simulink model "CACC_Center"  (R2022b)
settings: Solver=FixedStepAuto  StartTime=0.0  StopTime=Tsim  FixedStep=0.05  RelTol=1e-3
values from neighbouring files (symbols this model uses):
  h = 1.0    (= 1)    [ros_cacc.m]    (also in ros_cacc2.m)
  k1 = 1    [ros_cacc.m]    (also in ros_cacc2.m)
  k2 = 1    [ros_cacc.m]    (also in ros_cacc2.m)
  L = 0.32    [ros_cacc.m]    (also in ros_cacc2.m)
  r = 1    [ros_cacc.m]    (also in ros_cacc2.m)
  v_threshold = v_thr    (= 0.1)    [ros_cacc.m]    (also in ros_cacc2.m)
undefined symbols (not defined in the file or in its folder): angular, linear
libraries: ros2lib x7, robotcorelib x1
settings Model: VariantFading=off  Creator=harun  LastModifiedBy=harun
settings DataIOCC: ReturnWorkspaceOutputs=off
settings OptimizationCC: EnhancedBackFolding=on  PassReuseOutputArgsAs=Individual arguments  ZeroExternalMemoryAtStartup=off  ZeroInternalMemoryAtStartup=off  MaxStackSize=64  OptimizeBlockOrder=speed  DifferentSizesBufferReuse=on  OptimizationCustomize=off  EfficientTunableParamExpr=on
settings DebuggingCC: ParameterTunabilityLossMsg=error  UnconnectedInputMsg=warning  UnconnectedOutputMsg=warning  UnconnectedLineMsg=warning
settings HardwareCC: ProdBitPerLong=64  ProdHWDeviceType=Intel->x86-64 (Linux 64)
settings ModelReferenceCC: EnableRefExpFcnMdlSchedulingChecks=on
settings SFSimCC: MATLABDynamicMemAlloc=off
settings RTWCC: Description=Embedded Coder  SystemTargetFile=ert.tlc  HardwareBoard=Robot Operating System 2 (ROS 2)  TLCOptions="-aInlineSetEventsForThisBaseRateFcn=TLC_FALSE -aSuppressMultiTaskScheduler=TLC_FALSE  -aRateBasedStepFcn=0"  TemplateMakefile=ert_default_tmf  Toolchain=Colcon Tools  TargetLang=C++  DLArmComputeVersion=19.05
settings CodeAppCC: ForceParamTrailComments=on  IgnoreCustomStorageClasses=off  OperatorAnnotations=on  SimulinkDataObjDesc=on  SFDataObjDesc=on  InsertBlockDesc=on
settings ERTTargetCC: CodeInterfacePackaging=C++ class  SupportContinuousTime=on  SupportVariableSizeSignals=on  RootIOFormat=Structure reference

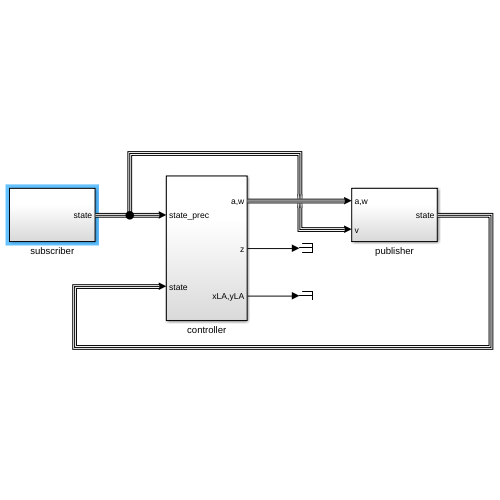
[thumbnail: Simulink's stored preview of the top-level diagram]
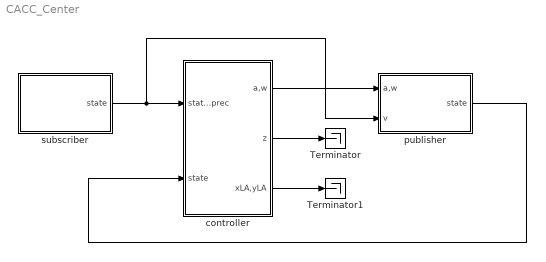
== system CACC_Center ==
  Terminator : Terminator
  Terminator1 : Terminator
  controller : Subsystem
  publisher : Subsystem
  subscriber : Subsystem
  wires:
  controller/3(xLA,yLA) -> Terminator1/1
  subscriber/1(state) -> publisher/2(v), controller/1(state_prec)
  publisher/1(state) -> controller/2(state)
  controller/1(a,w) -> publisher/1(a,w)
  controller/2(z) -> Terminator/1

== system CACC_Center/controller ==
  state_prec : Inport
  state : Inport  Port=2
  LA : Subsystem  TreatAsAtomicUnit=on
  a,w : Outport  VectorParamsAs1DForOutWhenUnconnected=off
  z : Outport  Port=2  VectorParamsAs1DForOutWhenUnconnected=off
  xLA,yLA : Outport  Port=3  VectorParamsAs1DForOutWhenUnconnected=off
  wires:
  state_prec/1 -> LA/1(state_prec)
  state/1 -> LA/2(state)
  LA/1(a,w) -> a,w/1
  LA/2(z) -> z/1
  LA/3(lookahead point) -> xLA,yLA/1

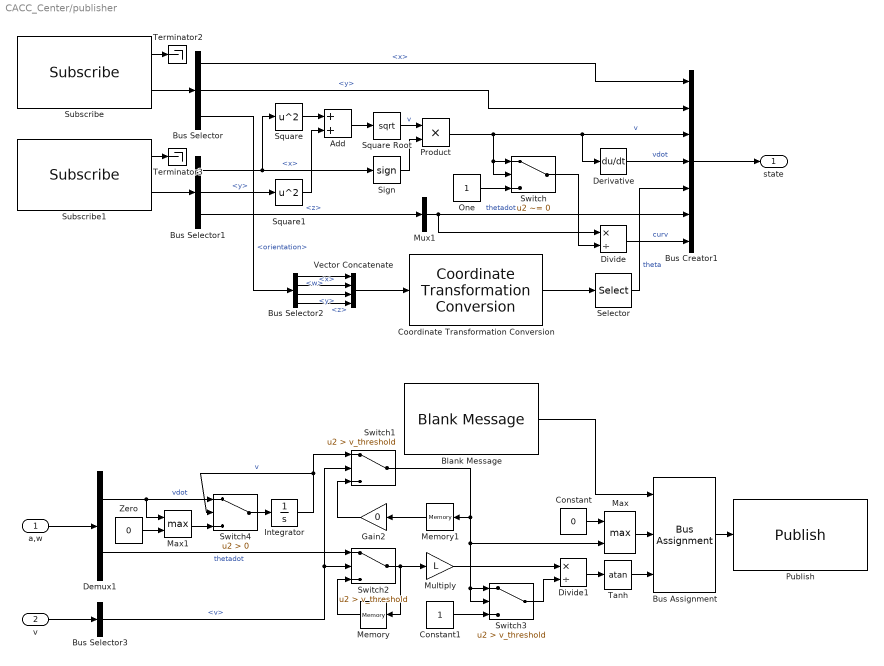
== system CACC_Center/publisher ==
  a,w : Inport
  v : Inport  Port=2
  Add : Sum
  Blank Message : ros2lib/Blank Message  messageClass=Message  entityType=geometry_msgs/Twist  messageType=geometry_msgs/Twist  SampleTime=0.05
  Bus Assignment : BusAssignment  AssignedSignals=linear.x,angular.z
  Bus Creator1 : BusCreator  Inputs=7
  Bus Selector : BusSelector  OutputSignals=pose.position.x,pose.position.y,pose.orientation
  Bus Selector1 : BusSelector  OutputSignals=twist.twist.linear.x,twist.twist.linear.y,twist.twist.angular.z
  Bus Selector2 : BusSelector  OutputSignals=w,x,y,z
  Bus Selector3 : BusSelector  OutputSignals=v
  Constant : Constant  Value=0
  Constant1 : Constant
  Coordinate Transformation Conversion : robotcorelib/Coordinate Transformation Conversion  InputRepresentation=Quaternion  InputEulerSequence=ZYX  ShowTrVecInputPort=on  OutputRepresentation=Euler Angles  OutputEulerSequence=ZYX  ShowTrVecOutputPort=on  SimulateUsing=Interpreted execution
  Demux1 : Demux  Outputs=2
  Derivative : Derivative
  Divide : Product  Inputs=*/
  Divide1 : Product  Inputs=*/
  Gain2 : Gain  Gain=0
  Integrator : Integrator  InitialCondition=0.0
  Max : MinMax  Function=max  Inputs=2
  Max1 : MinMax  Function=max  Inputs=2
  Memory : Memory
  Memory1 : Memory
  Multiply : Gain  Gain=L
  Mux1 : Mux  Inputs=1
  One : Constant  OutDataTypeStr=Inherit: Inherit via back propagation
  Product : Product
  Publish : ros2lib/Publish  topicSource=Specify your own  topic=cmd_vel  messageType=geometry_msgs/Twist  QOSHistory=Keep last  QOSDepth=1  QOSReliability=Reliable  QOSDurability=Volatile
  Selector : Selector  InputPortWidth=3  IndexOptions=Index vector (dialog)  Indices=[1]  OutputSizes=1
  Sign : Signum
  Square : Math  Operator=square
  Square Root : Sqrt
  Square1 : Math  Operator=square
  Subscribe : ros2lib/Subscribe  topicSource=Specify your own  topic=localization_pose  messageType=geometry_msgs/PoseStamped  sampleTime=0.1  QOSHistory=Keep last  QOSDepth=1  QOSReliability=Reliable  QOSDurability=Volatile
  Subscribe1 : ros2lib/Subscribe  topicSource=Specify your own  topic=odom  messageType=nav_msgs/Odometry  sampleTime=0.1  QOSHistory=Keep last  QOSDepth=1  QOSReliability=Reliable  QOSDurability=Volatile
  Switch : Switch  Criteria=u2 ~= 0  SaturateOnIntegerOverflow=off  InputSameDT=off
  Switch1 : Switch  Criteria=u2 > Threshold  Threshold=v_threshold  SaturateOnIntegerOverflow=off  InputSameDT=off
  Switch2 : Switch  Criteria=u2 > Threshold  Threshold=v_threshold  SaturateOnIntegerOverflow=off  InputSameDT=off
  Switch3 : Switch  Criteria=u2 > Threshold  Threshold=v_threshold  SaturateOnIntegerOverflow=off  InputSameDT=off
  Switch4 : Switch  Criteria=u2 > Threshold  SaturateOnIntegerOverflow=off  InputSameDT=off
  Tanh : Trigonometry  Operator=atan
  Terminator2 : Terminator
  Terminator3 : Terminator
  Vector Concatenate : Concatenate  NumInputs=4
  Zero : Constant  Value=0  OutDataTypeStr=Inherit: Inherit via back propagation
  state : Outport  VectorParamsAs1DForOutWhenUnconnected=off
  wires:
  Divide1/1 -> Tanh/1
  Mux1/1 -> Divide/1, Bus Creator1/6  "thetadot"
  Subscribe/1 -> Terminator2/1
  Subscribe/2 -> Bus Selector/1
  Subscribe1/2 -> Bus Selector1/1
  Subscribe1/1 -> Terminator3/1
  Memory1/1 -> Gain2/1
  Demux1/2 -> Switch2/1  "thetadot"
  Switch3/1 -> Divide1/2
  Memory/1 -> Switch2/3
  Switch/1 -> Divide/2
  Zero/1 -> Max1/2
  Divide/1 -> Bus Creator1/7  "curv"
  Selector/1 -> Bus Creator1/5  "theta"
  Switch2/1 -> Multiply/1, Memory/1
  Max1/1 -> Switch4/3
  Derivative/1 -> Bus Creator1/4  "vdot"
  Add/1 -> Square Root/1
  Integrator/1 -> Switch1/1, Switch4/2  "v"
  Bus Selector1/1 -> Square/1, Sign/1  "<x>"
  Square1/1 -> Add/2
  Square Root/1 -> Product/1  "v"
  Max/1 -> Bus Assignment/2
  Coordinate Transformation Conversion/1 -> Selector/1
  a,w/1 -> Demux1/1
  Bus Selector2/2 -> Vector Concatenate/2  "<x>"
  Product/1 -> Switch/1, Switch/2, Derivative/1, Bus Creator1/3  "v"
  Constant1/1 -> Switch3/3
  Bus Selector1/3 -> Mux1/1  "<z>"
  Demux1/1 -> Max1/1, Switch4/1  "vdot"
  Sign/1 -> Product/2
  Bus Selector2/1 -> Vector Concatenate/1  "<w>"
  Bus Assignment/1 -> Publish/1
  Bus Creator1/1 -> state/1
  Tanh/1 -> Bus Assignment/3
  Gain2/1 -> Switch1/3
  Blank Message/1 -> Bus Assignment/1
  Switch4/1 -> Integrator/1
  Bus Selector2/3 -> Vector Concatenate/3  "<y>"
  Switch1/1 -> Max/2, Switch3/1, Switch3/2, Memory1/1
  Vector Concatenate/1 -> Coordinate Transformation Conversion/1
  Bus Selector/3 -> Bus Selector2/1  "<orientation>"
  Constant/1 -> Max/1
  Square/1 -> Add/1
  Bus Selector/2 -> Bus Creator1/2  "<y>"
  Bus Selector3/1 -> Switch2/2, Switch1/2  "<v>"
  Bus Selector/1 -> Bus Creator1/1  "<x>"
  Bus Selector1/2 -> Square1/1  "<y>"
  One/1 -> Switch/3
  v/1 -> Bus Selector3/1
  Multiply/1 -> Divide1/1
  Bus Selector2/4 -> Vector Concatenate/4  "<z>"

== system CACC_Center/subscriber ==
  Bus Creator : BusCreator  Inputs=7
  Bus Selector : BusSelector  OutputSignals=x,y,v,vdot,theta,thetadot
  Derivative2 : Derivative
  Divide : Product  Inputs=*/
  One : Constant  OutDataTypeStr=Inherit: Inherit via back propagation
  Subscribe : ros2lib/Subscribe  topicSource=Specify your own  topic=cam_filtered  messageType=auna_its_msgs/CAM  sampleTime=0.1  QOSHistory=Keep last  QOSDepth=1  QOSReliability=Reliable  QOSDurability=Volatile
  Switch : Switch  Criteria=u2 ~= 0  SaturateOnIntegerOverflow=off  InputSameDT=off
  Terminator : Terminator
  Terminator4 : Terminator
  state : Outport  VectorParamsAs1DForOutWhenUnconnected=off
  wires:
  Subscribe/1 -> Terminator/1
  Subscribe/2 -> Bus Selector/1
  Bus Selector/4 -> Terminator4/1  "<vdot>"
  One/1 -> Switch/3
  Bus Selector/1 -> Bus Creator/1  "<x>"
  Bus Selector/2 -> Bus Creator/2  "<y>"
  Derivative2/1 -> Bus Creator/4  "vdot"
  Bus Selector/5 -> Bus Creator/5  "<theta>"
  Divide/1 -> Bus Creator/7  "curv"
  Bus Selector/3 -> Bus Creator/3, Derivative2/1, Switch/2, Switch/1  "<v>"
  Bus Creator/1 -> state/1
  Switch/1 -> Divide/2
  Bus Selector/6 -> Divide/1, Bus Creator/6  "<thetadot>"

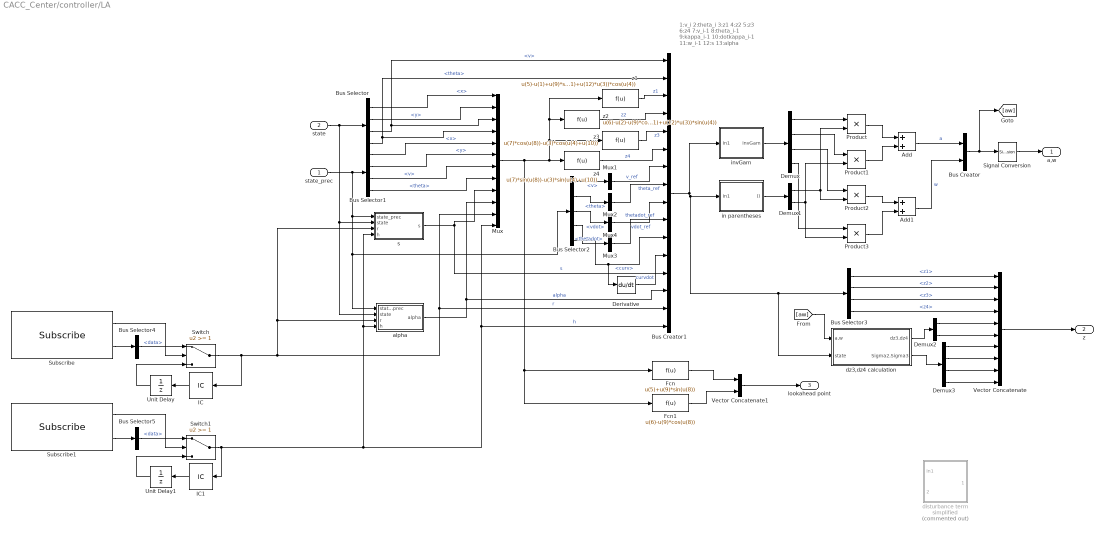
== system CACC_Center/controller/LA ==
  note: 1:v_i
      | 2:theta_i
      | 3:z1
      | 4:z2
      | 5:z3
      | 6:z4
      | 7:v_i-1
      | 8:theta_i-1
      | 9:kappa_i-1
      | 10:dotkappa_i-1
      | 11:w_i-1
      | 12:s
      | 13:alpha
  state_prec : Inport
  state : Inport  Port=2
  Add : Sum
  Add1 : Sum
  Bus Creator : BusCreator  Inputs=2
  Bus Creator1 : BusCreator  Inputs=16
  Bus Selector : BusSelector  OutputSignals=x,y,v,theta
  Bus Selector1 : BusSelector  OutputSignals=x,y,v,theta
  Bus Selector2 : BusSelector  OutputSignals=v,theta,vdot,thetadot,curv
  Bus Selector3 : BusSelector  OutputSignals=z1,z2,z3,z4
  Bus Selector4 : BusSelector  OutputSignals=data
  Bus Selector5 : BusSelector  OutputSignals=data
  Demux : Demux
  Demux1 : Demux  Outputs=2
  Demux2 : Demux  Outputs=2
  Demux3 : Demux
  Derivative : Derivative
  Fcn : Fcn  Expr=u(5)+u(9)*sin(u(8))
  Fcn1 : Fcn  Expr=u(6)-u(9)*cos(u(8))
  IC : InitialCondition  Value=r
  IC1 : InitialCondition  Value=h
  Mux : Mux  Inputs=12
  Mux{1..4} (4 alike) : Mux  Inputs=1
  Product{,1..3} (4 alike) : Product
  Signal Conversion : SignalConversion  OverrideOpt=off
  Subscribe : ros2lib/Subscribe  topicSource=Specify your own  topic=cacc/standstill_distance  messageType=example_interfaces/Float64  sampleTime=0.05  QOSHistory=Keep last  QOSDepth=1  QOSReliability=Reliable  QOSDurability=Volatile
      settings: LibrarySourceBlock=roslib/ROS 2/Subscribe
  Subscribe1 : ros2lib/Subscribe  topicSource=Specify your own  topic=cacc/time_gap  messageType=example_interfaces/Float64  sampleTime=0.05  QOSHistory=Keep last  QOSDepth=1  QOSReliability=Reliable  QOSDurability=Volatile
      settings: LibrarySourceBlock=roslib/ROS 2/Subscribe
  Switch : Switch  Threshold=1  SaturateOnIntegerOverflow=off  InputSameDT=off
  Switch1 : Switch  Threshold=1  SaturateOnIntegerOverflow=off  InputSameDT=off
  Unit Delay : UnitDelay  SampleTime=-1  HasFrameUpgradeWarning=on
  Unit Delay1 : UnitDelay  SampleTime=-1  HasFrameUpgradeWarning=on
  Vector Concatenate : Concatenate  NumInputs=10
  Vector Concatenate1 : Concatenate
  alpha : Subsystem
  disturbance term simplified : Subsystem  Commented=on
  dz3,dz4 calculation : Subsystem
  in parentheses : Subsystem
  invGam : Subsystem
  s : Subsystem
  z1 : Fcn  Expr=u(5)-u(1)+u(9)*sin(u(8))-(u(11)+u(12)*u(3))*cos(u(4))
  z2 : Fcn  Expr=u(6)-u(2)-u(9)*cos(u(8))-(u(11)+u(12)*u(3))*sin(u(4))
  z3 : Fcn  Expr=u(7)*cos(u(8))-u(3)*cos(u(4)+u(10))
  z4 : Fcn  Expr=u(7)*sin(u(8))-u(3)*sin(u(4)+u(10))
  a,w : Outport  VectorParamsAs1DForOutWhenUnconnected=off
  z : Outport  Port=2  VectorParamsAs1DForOutWhenUnconnected=off
  lookahead point : Outport  Port=3  VectorParamsAs1DForOutWhenUnconnected=off
  wires:
  Bus Selector/1 -> Mux/1  "<x>"
  Bus Selector/2 -> Mux/2  "<y>"
  Bus Selector/3 -> Bus Creator1/1, Mux/3  "<v>"
  Bus Selector/4 -> Bus Creator1/2, Mux/4  "<theta>"
  Bus Selector1/1 -> Mux/5  "<x>"
  Bus Selector1/2 -> Mux/6  "<y>"
  Bus Selector1/3 -> Mux/7  "<v>"
  Bus Selector1/4 -> Mux/8  "<theta>"
  Bus Creator/1 -> Signal Conversion/1, [aw]
  state/1 -> alpha/2(state), s/2(state), Bus Selector/1
  state_prec/1 -> alpha/1(state_prec), Bus Selector2/1, s/1(state_prec), Bus Selector1/1
  Mux/1 -> Fcn1/1, Fcn/1, z4/1, z1/1, z2/1, z3/1
  z1/1 -> Bus Creator1/3  "z1"
  z2/1 -> Bus Creator1/4  "z2"
  z3/1 -> Bus Creator1/5  "z3"
  z4/1 -> Bus Creator1/6  "z4"
  alpha/1(alpha) -> Bus Creator1/14, Mux/10  "alpha"
  s/1(s) -> Bus Creator1/13, Mux/9  "s"
  Bus Selector2/1 -> Mux1/1  "<v>"
  Bus Selector2/2 -> Mux2/1  "<theta>"
  Bus Selector2/5 -> Bus Creator1/11, Derivative/1  "<curv>"
  Derivative/1 -> Bus Creator1/12  "curvdot"
  Bus Selector2/4 -> Mux3/1  "<thetadot>"
  Bus Creator1/1 -> invGam/1(In1), dz3,dz4 calculation/2(state), Bus Selector3/1, in parentheses/1(In1)
  invGam/1(invGam) -> Demux/1
  Demux/1 -> Product/1
  in parentheses/1(()) -> Demux1/1
  Demux1/1 -> Product2/2, Product/2
  Demux/2 -> Product1/1
  Product/1 -> Add/1
  Product1/1 -> Add/2
  Demux/3 -> Product2/1
  Demux/4 -> Product3/1
  Demux1/2 -> Product1/2, Product3/2
  Product2/1 -> Add1/1
  Product3/1 -> Add1/2
  Add1/1 -> Bus Creator/2  "w"
  Mux1/1 -> Bus Creator1/7  "v_ref"
  Mux2/1 -> Bus Creator1/8  "theta_ref"
  Bus Selector3/1 -> Vector Concatenate/1  "<z1>"
  Bus Selector3/2 -> Vector Concatenate/2  "<z2>"
  Bus Selector3/3 -> Vector Concatenate/3  "<z3>"
  Bus Selector3/4 -> Vector Concatenate/4  "<z4>"
  Vector Concatenate/1 -> z/1
  Vector Concatenate1/1 -> lookahead point/1
  Fcn/1 -> Vector Concatenate1/1
  Fcn1/1 -> Vector Concatenate1/2
  dz3,dz4 calculation/1(dz3,dz4) -> Demux2/1
  [aw] -> dz3,dz4 calculation/1(a,w)
  Add/1 -> Bus Creator/1  "a"
  Demux2/1 -> Vector Concatenate/5
  Demux2/2 -> Vector Concatenate/6
  Signal Conversion/1 -> a,w/1
  Mux3/1 -> Bus Creator1/10  "thetadot_ref"
  Mux4/1 -> Bus Creator1/9  "vdot_ref"
  Bus Selector2/3 -> Mux4/1  "<vdot>"
  dz3,dz4 calculation/2(Sigma2,Sigma3) -> Demux3/1
  Demux3/1 -> Vector Concatenate/7
  Demux3/2 -> Vector Concatenate/8
  Demux3/3 -> Vector Concatenate/9
  Demux3/4 -> Vector Concatenate/10
  Subscribe/2 -> Bus Selector4/1
  Bus Selector4/1 -> Switch/1  "<data>"
  Subscribe/1 -> Switch/2
  Switch/1 -> s/3(r), alpha/3(r), Bus Creator1/15, Mux/11, IC/1  "r"
  IC/1 -> Unit Delay/1
  Unit Delay/1 -> Switch/3
  Unit Delay1/1 -> Switch1/3
  Bus Selector5/1 -> Switch1/1  "<data>"
  Subscribe1/2 -> Bus Selector5/1
  IC1/1 -> Unit Delay1/1
  Switch1/1 -> alpha/4(h), s/4(h), Bus Creator1/16, Mux/12, IC1/1  "h"
  Subscribe1/1 -> Switch1/2

== system CACC_Center/controller/LA/alpha ==
  state_prec : Inport
  state : Inport  Port=2
  r : Inport  Port=3
  h : Inport  Port=4
  Bus Selector : BusSelector  OutputSignals=curv
  Bus Selector1 : BusSelector  OutputSignals=v
  Fcn : Fcn  Expr=atan(u(1)*(u(3)+u(4)*u(2)))
  Mux : Mux
  alpha : Outport  VectorParamsAs1DForOutWhenUnconnected=off
  wires:
  state_prec/1 -> Bus Selector/1
  state/1 -> Bus Selector1/1
  Mux/1 -> Fcn/1
  Bus Selector/1 -> Mux/1  "<curv>"
  Bus Selector1/1 -> Mux/2  "<v>"
  Fcn/1 -> alpha/1
  r/1 -> Mux/3
  h/1 -> Mux/4

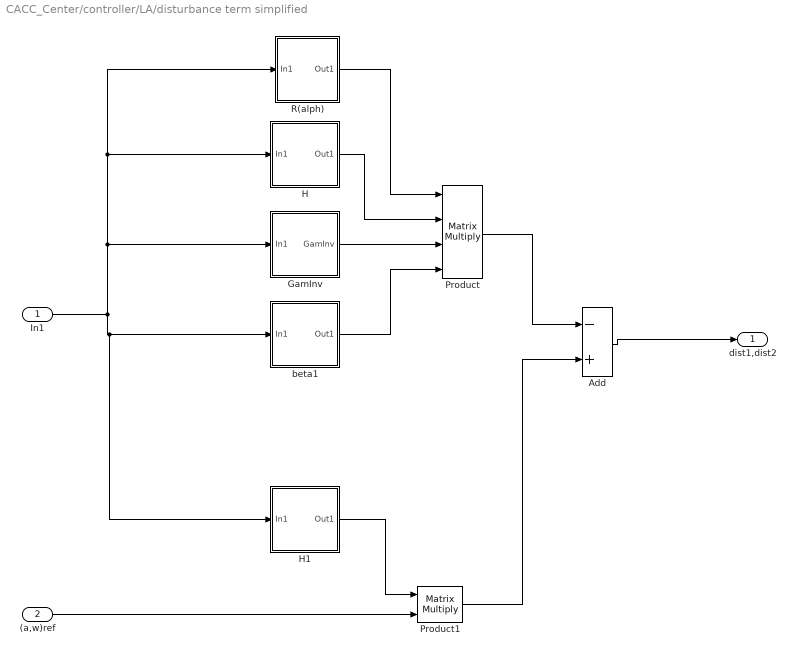
== system CACC_Center/controller/LA/disturbance term simplified ==
  In1 : Inport
  (a,w)ref : Inport  Port=2
  Add : Sum  Inputs=-+
  "GamInv " : Subsystem
  H : Subsystem
  H1 : Subsystem
  Product : Product  Inputs=4  Multiplication=Matrix(*)
  Product1 : Product  Multiplication=Matrix(*)
  R(alph) : Subsystem
  beta1 : Subsystem
  dist1,dist2 : Outport  VectorParamsAs1DForOutWhenUnconnected=off
  wires:
  Add/1 -> dist1,dist2/1
  Product/1 -> Add/1
  (a,w)ref/1 -> Product1/2
  H1/1(Out1) -> Product1/1
  beta1/1(Out1) -> Product/4
  "GamInv "/1(GamInv) -> Product/3
  H/1(Out1) -> Product/2
  R(alph)/1(Out1) -> Product/1
  In1/1 -> H/1(In1), R(alph)/1(In1), "GamInv "/1(In1), beta1/1(In1), H1/1(In1)
  Product1/1 -> Add/2

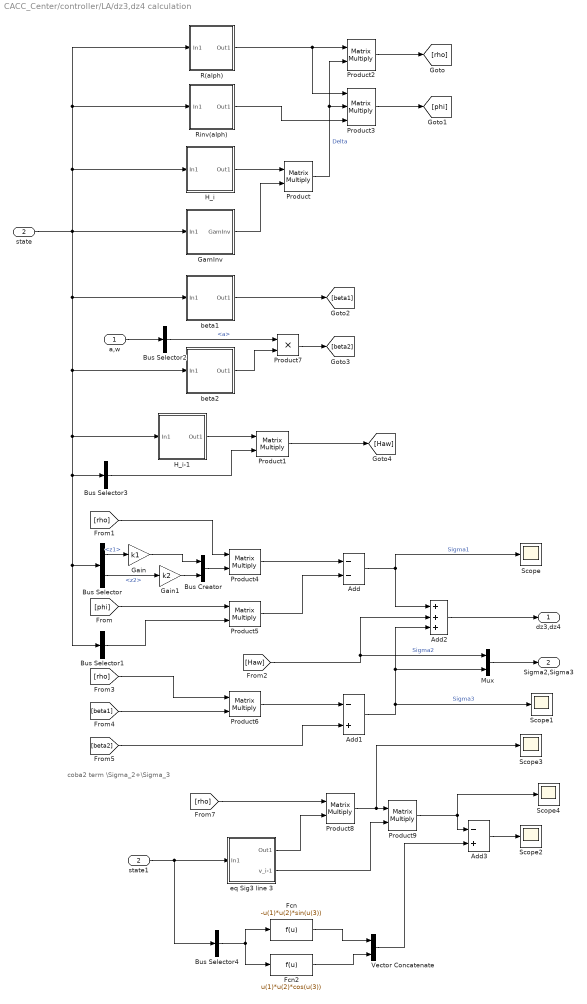
== system CACC_Center/controller/LA/dz3,dz4 calculation ==
  note: coba2 term \Sigma_2+\Sigma_3
  a,w : Inport
  state : Inport  Port=2
  Add : Sum  Inputs=--
  Add1 : Sum  Inputs=-+
  Add2 : Sum  Inputs=+++
  Add3 : Sum  Inputs=-+
  Bus Creator : BusCreator  Inputs=2
  Bus Selector : BusSelector  OutputSignals=z1,z2
  Bus Selector1 : BusSelector  OutputSignals=z3,z4  OutputAsBus=on
  Bus Selector2 : BusSelector  OutputSignals=a
  Bus Selector3 : BusSelector  OutputSignals=vdot_ref,thetadot_ref  OutputAsBus=on
  Bus Selector4 : BusSelector  OutputSignals=v_ref,thetadot_ref,theta_ref  OutputAsBus=on
  Fcn : Fcn  Expr=-u(1)*u(2)*sin(u(3))
  Fcn2 : Fcn  Expr=u(1)*u(2)*cos(u(3))
  Gain : Gain  Gain=k1
  Gain1 : Gain  Gain=k2
  "GamInv " : Subsystem
  H_i : Subsystem
  H_i-1 : Subsystem
  Mux : Mux  Inputs=2
  Product{,1..2,4..6,8..9} (8 alike) : Product  Multiplication=Matrix(*)
  Product3 : Product  Inputs=3  Multiplication=Matrix(*)
  Product7 : Product
  R(alph) : Subsystem
  Rinv(alph) : Subsystem
  Scope{,1..4} (5 alike) : Scope
  Vector Concatenate : Concatenate
  beta1 : Subsystem
  beta2 : Subsystem
  eq Sig3 line 3 : Subsystem
  state1 : InportShadow  Port=2
  dz3,dz4 : Outport  VectorParamsAs1DForOutWhenUnconnected=off
  Sigma2,Sigma3 : Outport  Port=2  VectorParamsAs1DForOutWhenUnconnected=off
  wires:
  state/1 -> beta1/1(In1), beta2/1(In1), H_i-1/1(In1), Bus Selector3/1, Bus Selector1/1, Bus Selector/1, Rinv(alph)/1(In1), R(alph)/1(In1), H_i/1(In1), "GamInv "/1(In1)
  H_i-1/1(Out1) -> Product1/1
  H_i/1(Out1) -> Product/1
  "GamInv "/1(GamInv) -> Product/2
  R(alph)/1(Out1) -> Product3/1, Product2/1
  Product/1 -> Product3/2, Product2/2  "Delta"
  Rinv(alph)/1(Out1) -> Product3/3
  Product2/1 -> [rho]
  Product3/1 -> [phi]
  beta1/1(Out1) -> [beta1]
  Product1/1 -> [Haw]
  Bus Selector/1 -> Gain/1  "<z1>"
  Bus Selector/2 -> Gain1/1  "<z2>"
  Gain/1 -> Bus Creator/1
  Gain1/1 -> Bus Creator/2
  Bus Creator/1 -> Product4/2
  [rho] -> Product4/1
  [phi] -> Product5/1
  Bus Selector1/1 -> Product5/2
  Product4/1 -> Add/1
  Product5/1 -> Add/2
  [rho] -> Product6/1
  [beta1] -> Product6/2
  Product6/1 -> Add1/1
  Add/1 -> Add2/1, Scope/1  "Sigma1"
  Add1/1 -> Mux/2, Add2/3, Scope1/1  "Sigma3"
  Add2/1 -> dz3,dz4/1
  a,w/1 -> Bus Selector2/1
  Bus Selector2/1 -> Product7/1  "<a>"
  [Haw] -> Mux/1, Add2/2  "Sigma2"
  Product7/1 -> [beta2]
  beta2/1(Out1) -> Product7/2
  [beta2] -> Add1/2
  Bus Selector3/1 -> Product1/2
  [rho] -> Product8/1
  eq Sig3 line 3/1(Out1) -> Product8/2
  Product8/1 -> Scope3/1, Product9/1
  Vector Concatenate/1 -> Add3/2
  Add3/1 -> Scope2/1
  state1/1 -> Bus Selector4/1, eq Sig3 line 3/1(In1)
  Bus Selector4/1 -> Fcn2/1, Fcn/1
  Fcn/1 -> Vector Concatenate/1
  Fcn2/1 -> Vector Concatenate/2
  eq Sig3 line 3/2(v_i-1) -> Product9/2
  Product9/1 -> Scope4/1, Add3/1
  Mux/1 -> Sigma2,Sigma3/1

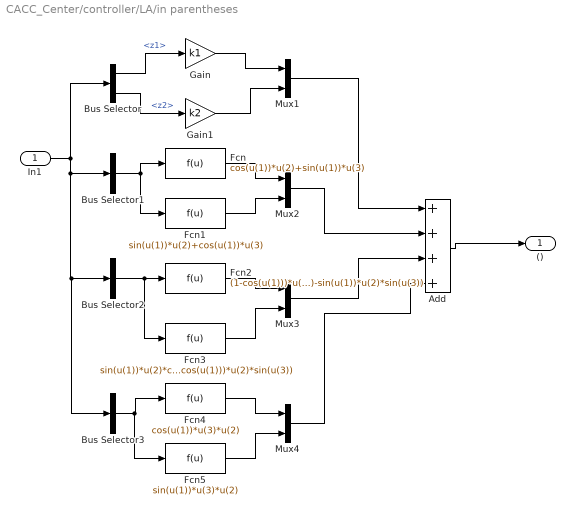
== system CACC_Center/controller/LA/in parentheses ==
  In1 : Inport
  Add : Sum  Inputs=++++
  Bus Selector : BusSelector  OutputSignals=z1,z2
  Bus Selector1 : BusSelector  OutputSignals=alpha,z3,z4  OutputAsBus=on
  Bus Selector2 : BusSelector  OutputSignals=alpha,v_ref,theta_ref  OutputAsBus=on
  Bus Selector3 : BusSelector  OutputSignals=theta_ref,thetadot_ref,s  OutputAsBus=on
  Fcn : Fcn  Expr=cos(u(1))*u(2)+sin(u(1))*u(3)
  Fcn1 : Fcn  Expr=sin(u(1))*u(2)+cos(u(1))*u(3)
  Fcn2 : Fcn  Expr=(1-cos(u(1)))*u(2)*cos(u(3))-sin(u(1))*u(2)*sin(u(3))
  Fcn3 : Fcn  Expr=sin(u(1))*u(2)*cos(u(3))+(1-cos(u(1)))*u(2)*sin(u(3))
  Fcn4 : Fcn  Expr=cos(u(1))*u(3)*u(2)
  Fcn5 : Fcn  Expr=sin(u(1))*u(3)*u(2)
  Gain : Gain  Gain=k1
  Gain1 : Gain  Gain=k2
  Mux{1..4} (4 alike) : Mux  Inputs=2
  () : Outport  VectorParamsAs1DForOutWhenUnconnected=off
  wires:
  In1/1 -> Bus Selector3/1, Bus Selector2/1, Bus Selector1/1, Bus Selector/1
  Bus Selector/1 -> Gain/1  "<z1>"
  Bus Selector/2 -> Gain1/1  "<z2>"
  Gain/1 -> Mux1/1
  Gain1/1 -> Mux1/2
  Bus Selector1/1 -> Fcn1/1, Fcn/1
  Fcn/1 -> Mux2/1
  Fcn1/1 -> Mux2/2
  Bus Selector2/1 -> Fcn3/1, Fcn2/1
  Fcn2/1 -> Mux3/1
  Fcn3/1 -> Mux3/2
  Bus Selector3/1 -> Fcn5/1, Fcn4/1
  Fcn4/1 -> Mux4/1
  Fcn5/1 -> Mux4/2
  Mux1/1 -> Add/1
  Mux2/1 -> Add/2
  Mux3/1 -> Add/3
  Mux4/1 -> Add/4
  Add/1 -> ()/1

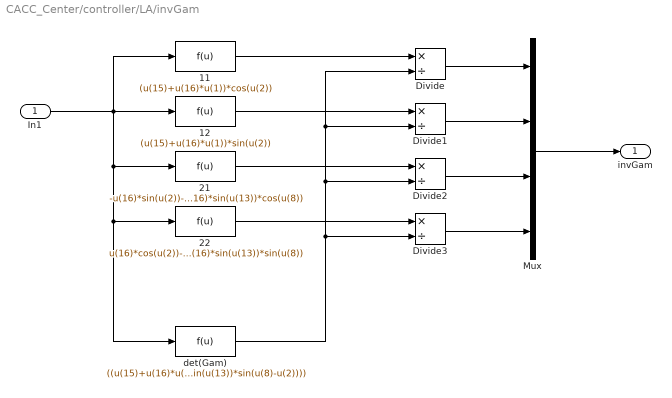
== system CACC_Center/controller/LA/invGam ==
  In1 : Inport
  11 : Fcn  Expr=(u(15)+u(16)*u(1))*cos(u(2))
  12 : Fcn  Expr=(u(15)+u(16)*u(1))*sin(u(2))
  21 : Fcn  Expr=-u(16)*sin(u(2))-u(16)*sin(u(13))*cos(u(8))
  22 : Fcn  Expr=u(16)*cos(u(2))-u(16)*sin(u(13))*sin(u(8))
  Divide{,1..3} (4 alike) : Product  Inputs=*/
  Mux : Mux
  det(Gam) : Fcn  Expr=((u(15)+u(16)*u(1))*(u(16)-u(16)*sin(u(13))*sin(u(8)-u(2))))
  invGam : Outport  VectorParamsAs1DForOutWhenUnconnected=off
  wires:
  In1/1 -> 11/1, 12/1, 22/1, det(Gam)/1, 21/1
  Mux/1 -> invGam/1
  11/1 -> Divide/1
  12/1 -> Divide1/1
  21/1 -> Divide2/1
  22/1 -> Divide3/1
  det(Gam)/1 -> Divide2/2, Divide1/2, Divide/2, Divide3/2
  Divide/1 -> Mux/1
  Divide1/1 -> Mux/2
  Divide2/1 -> Mux/3
  Divide3/1 -> Mux/4

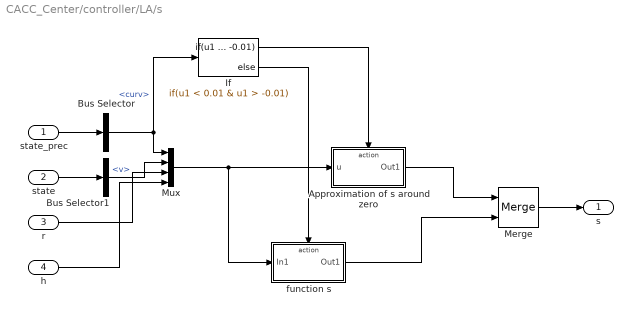
== system CACC_Center/controller/LA/s ==
  state_prec : Inport
  state : Inport  Port=2
  r : Inport  Port=3
  h : Inport  Port=4
  Approximation of s around zero : Subsystem  TreatAsAtomicUnit=on
  Bus Selector : BusSelector  OutputSignals=curv
  Bus Selector1 : BusSelector  OutputSignals=v
  If : If  IfExpression=u1 < 0.01 & u1 > -0.01
  Merge : Merge
  Mux : Mux
  function s : Subsystem  TreatAsAtomicUnit=on
  s : Outport  VectorParamsAs1DForOutWhenUnconnected=off
  wires:
  state_prec/1 -> Bus Selector/1
  Bus Selector/1 -> Mux/1, If/1  "<curv>"
  If/1 -> Approximation of s around zero/Action
  If/2 -> function s/Action
  Approximation of s around zero/1(Out1) -> Merge/1
  function s/1(Out1) -> Merge/2
  state/1 -> Bus Selector1/1
  Bus Selector1/1 -> Mux/2  "<v>"
  Mux/1 -> function s/1(In1), Approximation of s around zero/1(u)
  Merge/1 -> s/1
  r/1 -> Mux/3
  h/1 -> Mux/4

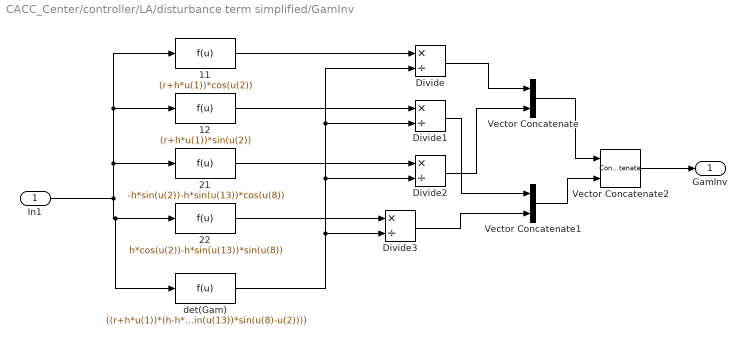
== system CACC_Center/controller/LA/disturbance term simplified/GamInv  ==
  In1 : Inport
  11 : Fcn  Expr=(r+h*u(1))*cos(u(2))
  12 : Fcn  Expr=(r+h*u(1))*sin(u(2))
  21 : Fcn  Expr=-h*sin(u(2))-h*sin(u(13))*cos(u(8))
  22 : Fcn  Expr=h*cos(u(2))-h*sin(u(13))*sin(u(8))
  Divide{,1..3} (4 alike) : Product  Inputs=*/
  Vector Concatenate : Concatenate
  Vector Concatenate1 : Concatenate
  Vector Concatenate2 : Concatenate  Mode=Multidimensional array  ConcatenateDimension=2
  det(Gam) : Fcn  Expr=((r+h*u(1))*(h-h*sin(u(13))*sin(u(8)-u(2))))
  GamInv : Outport  VectorParamsAs1DForOutWhenUnconnected=off
  wires:
  Vector Concatenate2/1 -> GamInv/1
  Vector Concatenate1/1 -> Vector Concatenate2/2
  Vector Concatenate/1 -> Vector Concatenate2/1
  Divide3/1 -> Vector Concatenate1/2
  Divide1/1 -> Vector Concatenate1/1
  Divide2/1 -> Vector Concatenate/2
  Divide/1 -> Vector Concatenate/1
  In1/1 -> 11/1, 12/1, 21/1, 22/1, det(Gam)/1
  det(Gam)/1 -> Divide3/2, Divide/2, Divide1/2, Divide2/2
  22/1 -> Divide3/1
  21/1 -> Divide2/1
  12/1 -> Divide1/1
  11/1 -> Divide/1

== system CACC_Center/controller/LA/disturbance term simplified/H ==
  In1 : Inport
  Bus Selector1 : BusSelector  OutputSignals=v,theta  OutputAsBus=on
  H11 : Fcn  Expr=cos(u(2))
  H12 : Fcn  Expr=-u(1)*sin(u(2))
  H21 : Fcn  Expr=sin(u(2))
  H22 : Fcn  Expr=u(1)*cos(u(2))
  Vector Concatenate3 : Concatenate
  Vector Concatenate4 : Concatenate
  Vector Concatenate5 : Concatenate  Mode=Multidimensional array  ConcatenateDimension=2
  Out1 : Outport  VectorParamsAs1DForOutWhenUnconnected=off
  wires:
  Vector Concatenate5/1 -> Out1/1
  H22/1 -> Vector Concatenate4/2
  H12/1 -> Vector Concatenate4/1
  H21/1 -> Vector Concatenate3/2
  H11/1 -> Vector Concatenate3/1
  Vector Concatenate4/1 -> Vector Concatenate5/2
  Vector Concatenate3/1 -> Vector Concatenate5/1
  In1/1 -> Bus Selector1/1
  Bus Selector1/1 -> H12/1, H21/1, H22/1, H11/1

== system CACC_Center/controller/LA/disturbance term simplified/H1 ==
  In1 : Inport
  Bus Selector1 : BusSelector  OutputSignals=v,theta  OutputAsBus=on
  H11 : Fcn  Expr=cos(u(2))
  H12 : Fcn  Expr=-u(1)*sin(u(2))
  H21 : Fcn  Expr=sin(u(2))
  H22 : Fcn  Expr=u(1)*cos(u(2))
  Vector Concatenate3 : Concatenate
  Vector Concatenate4 : Concatenate
  Vector Concatenate5 : Concatenate  Mode=Multidimensional array  ConcatenateDimension=2
  Out1 : Outport  VectorParamsAs1DForOutWhenUnconnected=off
  wires:
  Bus Selector1/1 -> H11/1, H22/1, H21/1, H12/1
  In1/1 -> Bus Selector1/1
  Vector Concatenate3/1 -> Vector Concatenate5/1
  Vector Concatenate4/1 -> Vector Concatenate5/2
  H11/1 -> Vector Concatenate3/1
  H21/1 -> Vector Concatenate3/2
  H12/1 -> Vector Concatenate4/1
  H22/1 -> Vector Concatenate4/2
  Vector Concatenate5/1 -> Out1/1

== system CACC_Center/controller/LA/disturbance term simplified/R(alph) ==
  In1 : Inport
  Bus Selector : BusSelector  OutputSignals=alpha
  R11 : Fcn  Expr=cos(u(1))
  R12 : Fcn  Expr=-sin(u(1))
  R21 : Fcn  Expr=sin(u(1))
  R22 : Fcn  Expr=cos(u(1))
  Vector Concatenate6 : Concatenate
  Vector Concatenate7 : Concatenate
  Vector Concatenate8 : Concatenate  Mode=Multidimensional array  ConcatenateDimension=2
  Out1 : Outport  VectorParamsAs1DForOutWhenUnconnected=off
  wires:
  Vector Concatenate8/1 -> Out1/1
  R22/1 -> Vector Concatenate7/2
  R12/1 -> Vector Concatenate7/1
  R21/1 -> Vector Concatenate6/2
  R11/1 -> Vector Concatenate6/1
  Vector Concatenate7/1 -> Vector Concatenate8/2
  Vector Concatenate6/1 -> Vector Concatenate8/1
  Bus Selector/1 -> R22/1, R21/1, R12/1, R11/1  "<alpha>"
  In1/1 -> Bus Selector/1

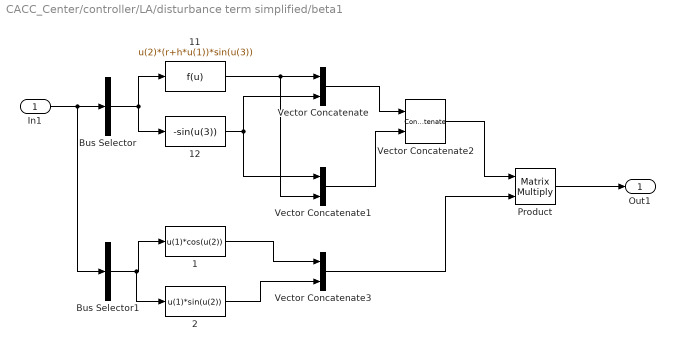
== system CACC_Center/controller/LA/disturbance term simplified/beta1 ==
  In1 : Inport
  1 : Fcn  Expr=u(1)*cos(u(2))
  11 : Fcn  Expr=u(2)*(r+h*u(1))*sin(u(3))
  12 : Fcn  Expr=-sin(u(3))
  2 : Fcn  Expr=u(1)*sin(u(2))
  Bus Selector : BusSelector  OutputSignals=v,curv,alpha  OutputAsBus=on
  Bus Selector1 : BusSelector  OutputSignals=v_ref,theta_ref  OutputAsBus=on
  Product : Product  Multiplication=Matrix(*)
  Vector Concatenate : Concatenate
  Vector Concatenate1 : Concatenate
  Vector Concatenate2 : Concatenate  Mode=Multidimensional array  ConcatenateDimension=2
  Vector Concatenate3 : Concatenate
  Out1 : Outport  VectorParamsAs1DForOutWhenUnconnected=off
  wires:
  In1/1 -> Bus Selector1/1, Bus Selector/1
  Bus Selector/1 -> 11/1, 12/1
  11/1 -> Vector Concatenate1/2, Vector Concatenate/1
  12/1 -> Vector Concatenate1/1, Vector Concatenate/2
  Vector Concatenate/1 -> Vector Concatenate2/1
  Vector Concatenate1/1 -> Vector Concatenate2/2
  1/1 -> Vector Concatenate3/1
  2/1 -> Vector Concatenate3/2
  Bus Selector1/1 -> 2/1, 1/1
  Vector Concatenate2/1 -> Product/1
  Vector Concatenate3/1 -> Product/2
  Product/1 -> Out1/1

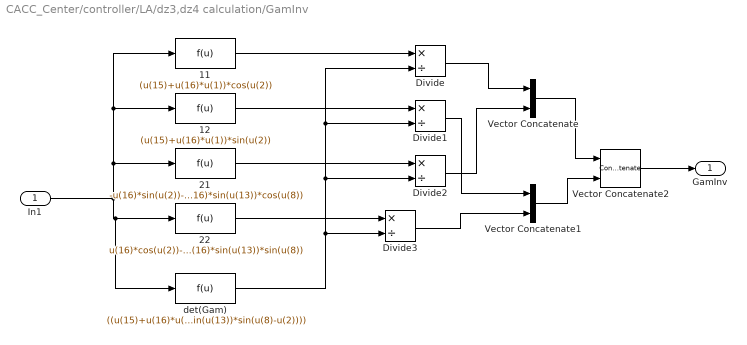
== system CACC_Center/controller/LA/dz3,dz4 calculation/GamInv  ==
  In1 : Inport
  11 : Fcn  Expr=(u(15)+u(16)*u(1))*cos(u(2))
  12 : Fcn  Expr=(u(15)+u(16)*u(1))*sin(u(2))
  21 : Fcn  Expr=-u(16)*sin(u(2))-u(16)*sin(u(13))*cos(u(8))
  22 : Fcn  Expr=u(16)*cos(u(2))-u(16)*sin(u(13))*sin(u(8))
  Divide{,1..3} (4 alike) : Product  Inputs=*/
  Vector Concatenate : Concatenate
  Vector Concatenate1 : Concatenate
  Vector Concatenate2 : Concatenate  Mode=Multidimensional array  ConcatenateDimension=2
  det(Gam) : Fcn  Expr=((u(15)+u(16)*u(1))*(u(16)-u(16)*sin(u(13))*sin(u(8)-u(2))))
  GamInv : Outport  VectorParamsAs1DForOutWhenUnconnected=off
  wires:
  11/1 -> Divide/1
  12/1 -> Divide1/1
  21/1 -> Divide2/1
  22/1 -> Divide3/1
  det(Gam)/1 -> Divide2/2, Divide1/2, Divide/2, Divide3/2
  In1/1 -> det(Gam)/1, 22/1, 21/1, 12/1, 11/1
  Divide/1 -> Vector Concatenate/1
  Divide2/1 -> Vector Concatenate/2
  Divide1/1 -> Vector Concatenate1/1
  Divide3/1 -> Vector Concatenate1/2
  Vector Concatenate/1 -> Vector Concatenate2/1
  Vector Concatenate1/1 -> Vector Concatenate2/2
  Vector Concatenate2/1 -> GamInv/1

== system CACC_Center/controller/LA/dz3,dz4 calculation/H_i ==
  In1 : Inport
  Bus Selector1 : BusSelector  OutputSignals=v,theta  OutputAsBus=on
  H11 : Fcn  Expr=cos(u(2))
  H12 : Fcn  Expr=-u(1)*sin(u(2))
  H21 : Fcn  Expr=sin(u(2))
  H22 : Fcn  Expr=u(1)*cos(u(2))
  Vector Concatenate3 : Concatenate
  Vector Concatenate4 : Concatenate
  Vector Concatenate5 : Concatenate  Mode=Multidimensional array  ConcatenateDimension=2
  Out1 : Outport  VectorParamsAs1DForOutWhenUnconnected=off
  wires:
  Bus Selector1/1 -> H11/1, H22/1, H21/1, H12/1
  In1/1 -> Bus Selector1/1
  Vector Concatenate3/1 -> Vector Concatenate5/1
  Vector Concatenate4/1 -> Vector Concatenate5/2
  H11/1 -> Vector Concatenate3/1
  H21/1 -> Vector Concatenate3/2
  H12/1 -> Vector Concatenate4/1
  H22/1 -> Vector Concatenate4/2
  Vector Concatenate5/1 -> Out1/1

== system CACC_Center/controller/LA/dz3,dz4 calculation/H_i-1 ==
  In1 : Inport
  Bus Selector1 : BusSelector  OutputSignals=v_ref,theta_ref  OutputAsBus=on
  H11 : Fcn  Expr=cos(u(2))
  H12 : Fcn  Expr=-u(1)*sin(u(2))
  H21 : Fcn  Expr=sin(u(2))
  H22 : Fcn  Expr=u(1)*cos(u(2))
  Vector Concatenate3 : Concatenate
  Vector Concatenate4 : Concatenate
  Vector Concatenate5 : Concatenate  Mode=Multidimensional array  ConcatenateDimension=2
  Out1 : Outport  VectorParamsAs1DForOutWhenUnconnected=off
  wires:
  Vector Concatenate5/1 -> Out1/1
  H22/1 -> Vector Concatenate4/2
  H12/1 -> Vector Concatenate4/1
  H21/1 -> Vector Concatenate3/2
  H11/1 -> Vector Concatenate3/1
  Vector Concatenate4/1 -> Vector Concatenate5/2
  Vector Concatenate3/1 -> Vector Concatenate5/1
  In1/1 -> Bus Selector1/1
  Bus Selector1/1 -> H12/1, H21/1, H22/1, H11/1

== system CACC_Center/controller/LA/dz3,dz4 calculation/R(alph) ==
  In1 : Inport
  Bus Selector : BusSelector  OutputSignals=alpha
  R11 : Fcn  Expr=cos(u(1))
  R12 : Fcn  Expr=-sin(u(1))
  R21 : Fcn  Expr=sin(u(1))
  R22 : Fcn  Expr=cos(u(1))
  Vector Concatenate6 : Concatenate
  Vector Concatenate7 : Concatenate
  Vector Concatenate8 : Concatenate  Mode=Multidimensional array  ConcatenateDimension=2
  Out1 : Outport  VectorParamsAs1DForOutWhenUnconnected=off
  wires:
  In1/1 -> Bus Selector/1
  Bus Selector/1 -> R11/1, R12/1, R21/1, R22/1  "<alpha>"
  Vector Concatenate6/1 -> Vector Concatenate8/1
  Vector Concatenate7/1 -> Vector Concatenate8/2
  R11/1 -> Vector Concatenate6/1
  R21/1 -> Vector Concatenate6/2
  R12/1 -> Vector Concatenate7/1
  R22/1 -> Vector Concatenate7/2
  Vector Concatenate8/1 -> Out1/1

== system CACC_Center/controller/LA/dz3,dz4 calculation/Rinv(alph) ==
  In1 : Inport
  Bus Selector : BusSelector  OutputSignals=alpha
  R11 : Fcn  Expr=cos(u(1))
  R12 : Fcn  Expr=sin(u(1))
  R21 : Fcn  Expr=-sin(u(1))
  R22 : Fcn  Expr=cos(u(1))
  Vector Concatenate6 : Concatenate
  Vector Concatenate7 : Concatenate
  Vector Concatenate8 : Concatenate  Mode=Multidimensional array  ConcatenateDimension=2
  Out1 : Outport  VectorParamsAs1DForOutWhenUnconnected=off
  wires:
  Vector Concatenate8/1 -> Out1/1
  R22/1 -> Vector Concatenate7/2
  R12/1 -> Vector Concatenate7/1
  R21/1 -> Vector Concatenate6/2
  R11/1 -> Vector Concatenate6/1
  Vector Concatenate7/1 -> Vector Concatenate8/2
  Vector Concatenate6/1 -> Vector Concatenate8/1
  Bus Selector/1 -> R22/1, R21/1, R12/1, R11/1  "<alpha>"
  In1/1 -> Bus Selector/1

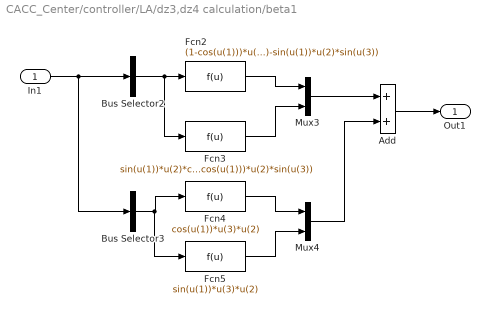
== system CACC_Center/controller/LA/dz3,dz4 calculation/beta1 ==
  In1 : Inport
  Add : Sum
  Bus Selector2 : BusSelector  OutputSignals=alpha,v_ref,theta_ref  OutputAsBus=on
  Bus Selector3 : BusSelector  OutputSignals=theta_ref,thetadot_ref,s  OutputAsBus=on
  Fcn2 : Fcn  Expr=(1-cos(u(1)))*u(2)*cos(u(3))-sin(u(1))*u(2)*sin(u(3))
  Fcn3 : Fcn  Expr=sin(u(1))*u(2)*cos(u(3))+(1-cos(u(1)))*u(2)*sin(u(3))
  Fcn4 : Fcn  Expr=cos(u(1))*u(3)*u(2)
  Fcn5 : Fcn  Expr=sin(u(1))*u(3)*u(2)
  Mux3 : Mux  Inputs=2
  Mux4 : Mux  Inputs=2
  Out1 : Outport  VectorParamsAs1DForOutWhenUnconnected=off
  wires:
  Bus Selector2/1 -> Fcn3/1, Fcn2/1
  Fcn2/1 -> Mux3/1
  Fcn3/1 -> Mux3/2
  Bus Selector3/1 -> Fcn5/1, Fcn4/1
  Fcn4/1 -> Mux4/1
  Fcn5/1 -> Mux4/2
  Mux3/1 -> Add/1
  Mux4/1 -> Add/2
  In1/1 -> Bus Selector3/1, Bus Selector2/1
  Add/1 -> Out1/1

== system CACC_Center/controller/LA/dz3,dz4 calculation/beta2 ==
  In1 : Inport
  Bus Selector : BusSelector  OutputSignals=v,theta,alpha,curv,r,h  OutputAsBus=on
  Mux : Mux  Inputs=2
  beta2_1 : Fcn  Expr=-u(1)*sin(u(2)+u(3))*(u(6)*u(4)*cos(u(3))^2)
  beta2_2 : Fcn  Expr=u(1)*cos(u(2)+u(3))*(u(6)*u(4)*cos(u(3))^2)
  Out1 : Outport  VectorParamsAs1DForOutWhenUnconnected=off
  wires:
  In1/1 -> Bus Selector/1
  Bus Selector/1 -> beta2_2/1, beta2_1/1
  beta2_1/1 -> Mux/1
  beta2_2/1 -> Mux/2
  Mux/1 -> Out1/1

== system CACC_Center/controller/LA/dz3,dz4 calculation/eq Sig3 line 3 ==
  In1 : Inport
  1 : Fcn  Expr=u(1)*cos(u(2))
  2 : Fcn  Expr=u(1)*sin(u(2))
  Bus Selector1 : BusSelector  OutputSignals=v_ref,theta_ref  OutputAsBus=on
  Vector Concatenate3 : Concatenate
  mat : Subsystem
  Out1 : Outport  VectorParamsAs1DForOutWhenUnconnected=off
  v_i-1 : Outport  Port=2  VectorParamsAs1DForOutWhenUnconnected=off
  wires:
  In1/1 -> mat/1(In1), Bus Selector1/1
  Bus Selector1/1 -> 2/1, 1/1
  1/1 -> Vector Concatenate3/1
  2/1 -> Vector Concatenate3/2
  mat/1(Out1) -> Out1/1
  Vector Concatenate3/1 -> v_i-1/1

== system CACC_Center/controller/LA/s/Approximation of s around zero ==
  u : Inport
  Action Port : ActionPort  ActionPortLabel=if(u1 < 0.01 & u1 > -0.01)
  Taylor approximation 3rd order : Fcn  Expr=0.5*(u(3)+u(4)*u(2))^2*u(1)-0.125*(u(3)+u(4)*u(2))^4*u(1)^3
  Out1 : Outport  VectorParamsAs1DForOutWhenUnconnected=off
  wires:
  u/1 -> Taylor approximation 3rd order/1
  Taylor approximation 3rd order/1 -> Out1/1

== system CACC_Center/controller/LA/s/function s ==
  In1 : Inport
  Action Port : ActionPort  ActionPortLabel=else
  function s : Fcn  Expr=(-1+sqrt(1+u(1)^2*(u(3)+u(4)*u(2))^2))/u(1)
  Out1 : Outport  VectorParamsAs1DForOutWhenUnconnected=off
  wires:
  In1/1 -> function s/1
  function s/1 -> Out1/1

== system CACC_Center/controller/LA/dz3,dz4 calculation/eq Sig3 line 3/mat ==
  In1 : Inport
  Bus Selector : BusSelector  OutputSignals=curv,v,alpha,r,h  OutputAsBus=on
  R11 : Fcn  Expr=u(1)*(u(4)+u(5)*u(2))*sin(u(3))
  R12 : Fcn  Expr=-sin(u(3))
  R21 : Fcn  Expr=sin(u(3))
  R22 : Fcn  Expr=u(1)*(u(4)+u(5)*u(2))*sin(u(3))
  Vector Concatenate6 : Concatenate
  Vector Concatenate7 : Concatenate
  Vector Concatenate8 : Concatenate  Mode=Multidimensional array  ConcatenateDimension=2
  Out1 : Outport  VectorParamsAs1DForOutWhenUnconnected=off
  wires:
  Vector Concatenate8/1 -> Out1/1
  R22/1 -> Vector Concatenate7/2
  R12/1 -> Vector Concatenate7/1
  R21/1 -> Vector Concatenate6/2
  R11/1 -> Vector Concatenate6/1
  Vector Concatenate7/1 -> Vector Concatenate8/2
  Vector Concatenate6/1 -> Vector Concatenate8/1
  Bus Selector/1 -> R12/1, R21/1, R22/1, R11/1
  In1/1 -> Bus Selector/1
